simulink model "NetraAI_DigitalTwin_V1"  (Simulink 8.3)
settings: Solver=FixedStepDiscrete  StartTime=0.0  StopTime=300  RelTol=1e-3
Description:
  | ANEYE / NetraAI TRACE-DR Digital Twin V1. Arrival period and fundus capture time are assumptions. AI service time 8.67151 s is a measured single-reference-case engineering value. TRACE routeCode is generated by the MATLAB trust engine. This model is a research engineering prototype and not clinical validation.
settings Model: Creator=kaustav  LastModifiedBy=kaustav
settings DataIOCC: SignalLoggingSaveFormat=Dataset
settings DebuggingCC: UnderspecifiedInitializationDetection=Simplified  StateNameClashWarn=none
settings GRTTargetCC: CombineOutputUpdateFcns=on  GRTInterface=off

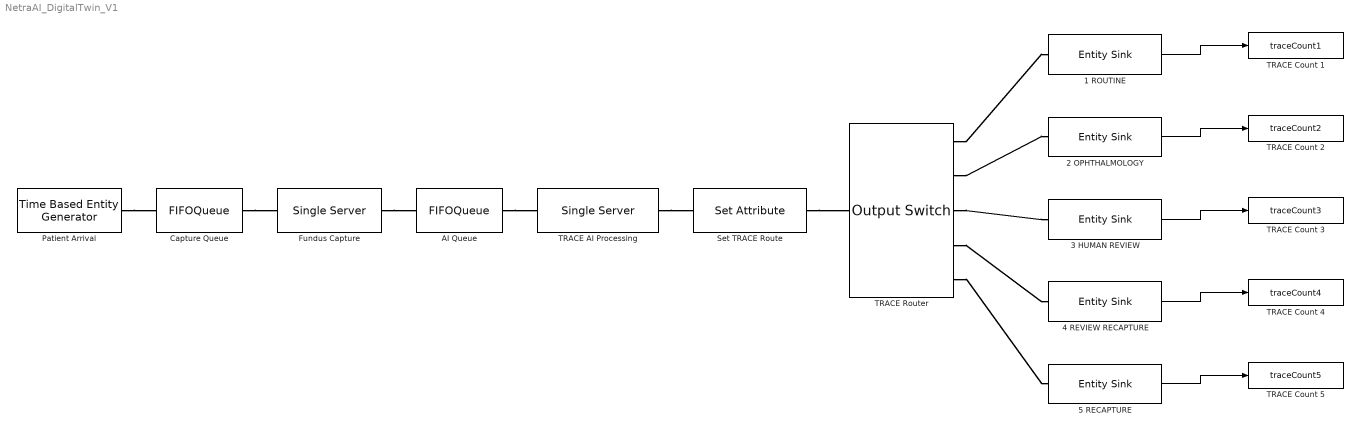
== system NetraAI_DigitalTwin_V1 ==
  1 ROUTINE : EntitySink  StatNumberArrived=on
  2 OPHTHALMOLOGY : EntitySink  StatNumberArrived=on
  3 HUMAN REVIEW : EntitySink  StatNumberArrived=on
  4 REVIEW RECAPTURE : EntitySink  StatNumberArrived=on
  5 RECAPTURE : EntitySink  StatNumberArrived=on
  AI Queue : FIFOQueue  Capacity=100
  Capture Queue : FIFOQueue  Capacity=100
  Fundus Capture : SingleServer  ServiceTime=12
  Patient Arrival : TimeBasedEntityGenerator  Period=15
  Set TRACE Route : SetAttribute  AttributeName=routeCode  AttributeValue=2  EvaluatedAttributeValue={ 2}
  TRACE AI Processing : SingleServer  ServiceTime=8.67151
  TRACE Count 1 : ToWorkspace  VariableName=traceCount1  SampleTime=-1
  TRACE Count 2 : ToWorkspace  VariableName=traceCount2  SampleTime=-1
  TRACE Count 3 : ToWorkspace  VariableName=traceCount3  SampleTime=-1
  TRACE Count 4 : ToWorkspace  VariableName=traceCount4  SampleTime=-1
  TRACE Count 5 : ToWorkspace  VariableName=traceCount5  SampleTime=-1
  TRACE Router : OutputSwitch  NumberOutputPorts=5  SwitchingCriterion=From attribute  AttributeName=routeCode
  wires:
  1 ROUTINE/1 -> TRACE Count 1/1
  2 OPHTHALMOLOGY/1 -> TRACE Count 2/1
  3 HUMAN REVIEW/1 -> TRACE Count 3/1
  4 REVIEW RECAPTURE/1 -> TRACE Count 4/1
  5 RECAPTURE/1 -> TRACE Count 5/1
  connections:
  Patient Arrival/RConn1 -- Capture Queue/LConn1
  Capture Queue/RConn1 -- Fundus Capture/LConn1
  Fundus Capture/RConn1 -- AI Queue/LConn1
  AI Queue/RConn1 -- TRACE AI Processing/LConn1
  TRACE AI Processing/RConn1 -- Set TRACE Route/LConn1
  Set TRACE Route/RConn1 -- TRACE Router/LConn1
  TRACE Router/RConn1 -- 1 ROUTINE/LConn1
  TRACE Router/RConn2 -- 2 OPHTHALMOLOGY/LConn1
  TRACE Router/RConn3 -- 3 HUMAN REVIEW/LConn1
  TRACE Router/RConn4 -- 4 REVIEW RECAPTURE/LConn1
  TRACE Router/RConn5 -- 5 RECAPTURE/LConn1
